simulink model "Function_Call_Subsystem_Ex"  (R2021b)
settings: Solver=VariableStepAuto  StartTime=0.0  StopTime=10.0  RelTol=1e-3
libraries: simulink x11
settings Model: Creator=t  LastModifiedBy=t

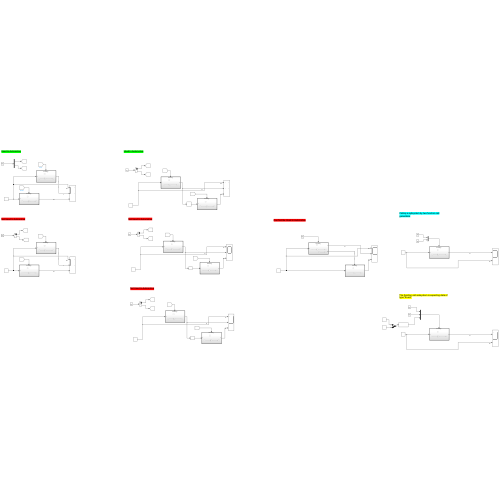
[thumbnail: Simulink's stored preview of the top-level diagram]
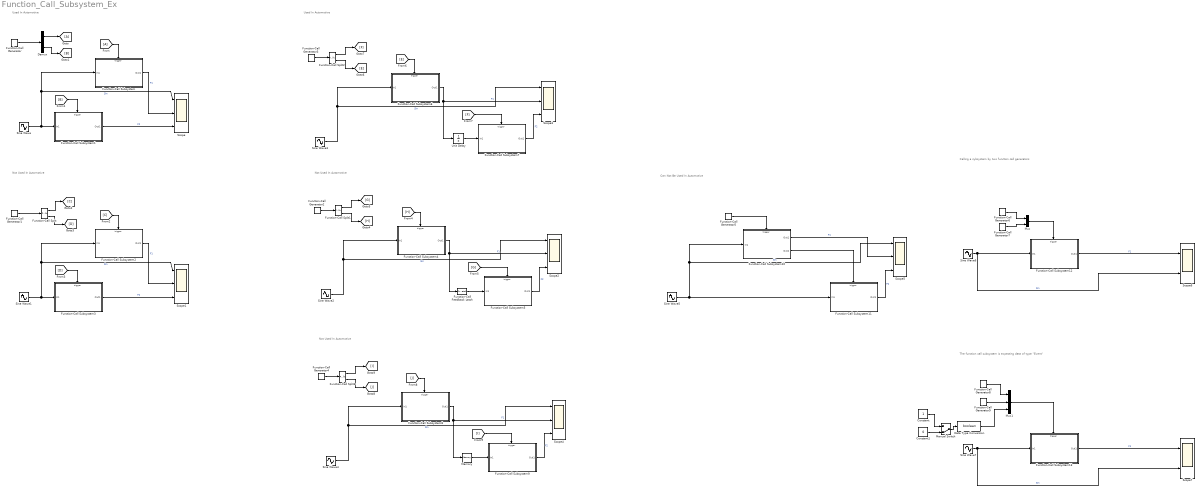
== system Function_Call_Subsystem_Ex ==
  note: Used In Automotive
  note: Not Used In Automotive
  note: Used In Automotive
  note: Not Used In Automotive
  note: Not Used In Automotive
  note: Can Not Be Used In Automotive
  note: Calling a sybsystem by two function call generators
  note: The function call subsystem is expecting data of type "Event"
  Constant : Constant
  Constant1 : Constant  Value=0
  Data Type Conversion : DataTypeConversion  OutDataTypeStr=boolean
  Demux : Demux  Outputs=2
  Function-Call Feedback Latch : FunctionCallFeedbackLatch
  Function-Call Generator{,1..6,8} (8 alike) : simulink/Ports & Subsystems/Function-Call Generator  sample_time=0.2  numberOfIterations=1  DisallowWideOutput=off
  Function-Call Generator7 : simulink/Ports & Subsystems/Function-Call Generator  sample_time=0.5  numberOfIterations=1  DisallowWideOutput=off
  Function-Call Generator9 : simulink/Ports & Subsystems/Function-Call Generator  sample_time=0.5  numberOfIterations=1  DisallowWideOutput=off
  Function-Call Split{,1..3} (4 alike) : FunctionCallSplit  IconShape=distinctive  NumOutputPorts=2  OutputPortLayout=default
  Function-Call Subsystem : Subsystem  TreatAsAtomicUnit=on
  Function-Call Subsystem1 : Subsystem  TreatAsAtomicUnit=on
  Function-Call Subsystem10 : Subsystem  TreatAsAtomicUnit=on
  Function-Call Subsystem11 : Subsystem  TreatAsAtomicUnit=on
  Function-Call Subsystem12 : Subsystem  TreatAsAtomicUnit=on
  Function-Call Subsystem13 : Subsystem  TreatAsAtomicUnit=on
  Function-Call Subsystem2 : Subsystem  TreatAsAtomicUnit=on
  Function-Call Subsystem3 : Subsystem  TreatAsAtomicUnit=on
  Function-Call Subsystem4 : Subsystem  TreatAsAtomicUnit=on
  Function-Call Subsystem5 : Subsystem  TreatAsAtomicUnit=on
  Function-Call Subsystem6 : Subsystem  TreatAsAtomicUnit=on
  Function-Call Subsystem7 : Subsystem  TreatAsAtomicUnit=on
  Function-Call Subsystem8 : Subsystem  TreatAsAtomicUnit=on
  Function-Call Subsystem9 : Subsystem  TreatAsAtomicUnit=on
  Manual Switch : ManualSwitch  CurrentSetting=0
  Memory : Memory
  Mux : Mux  Inputs=2
  Mux1 : Mux  Inputs=3
  Scope{,1..5} (6 alike) : Scope  NumInputPorts=3
  Scope6 : Scope  NumInputPorts=2
  Scope7 : Scope  NumInputPorts=2
  Sine Wave{,1..7} (8 alike) : Sin  SampleTime=0.1
  Unit Delay : UnitDelay  SampleTime=-1  HasFrameUpgradeWarning=on
  wires:
  Function-Call Generator/1 -> Demux/1
  Sine Wave/1 -> Scope/1, Function-Call Subsystem/1(In1), Function-Call Subsystem1/1(In1)  "Sin"
  Function-Call Subsystem/1(Out1) -> Scope/2  "F1"
  Function-Call Subsystem1/1(Out1) -> Scope/3  "F2"
  Demux/1 -> [A]
  Demux/2 -> [B]
  [A] -> Function-Call Subsystem/Trigger
  [B] -> Function-Call Subsystem1/Trigger
  Function-Call Subsystem3/1(Out1) -> Scope1/3  "F2"
  Function-Call Subsystem2/1(Out1) -> Scope1/2  "F1"
  Sine Wave1/1 -> Function-Call Subsystem3/1(In1), Function-Call Subsystem2/1(In1), Scope1/1  "Sin"
  Function-Call Generator1/1 -> Function-Call Split/1
  Function-Call Split/1 -> [C]
  [C] -> Function-Call Subsystem2/Trigger
  Function-Call Split/2 -> [D]
  [D] -> Function-Call Subsystem3/Trigger
  [G] -> Function-Call Subsystem5/Trigger
  [H] -> Function-Call Subsystem4/Trigger
  Function-Call Subsystem5/1(Out1) -> Scope2/3  "F2"
  Function-Call Subsystem4/1(Out1) -> Scope2/2, Function-Call Feedback Latch/1  "F1"
  Sine Wave2/1 -> Function-Call Subsystem4/1(In1), Scope2/1  "Sin"
  Function-Call Generator2/1 -> Function-Call Split1/1
  Function-Call Split1/2 -> [H]
  Function-Call Split1/1 -> [G]
  Function-Call Feedback Latch/1 -> Function-Call Subsystem5/1(In1)
  Unit Delay/1 -> Function-Call Subsystem7/1(In1)
  Function-Call Split2/1 -> [F]
  Function-Call Split2/2 -> [E]
  Function-Call Generator3/1 -> Function-Call Split2/1
  Sine Wave3/1 -> Scope3/1, Function-Call Subsystem6/1(In1)  "Sin"
  Function-Call Subsystem6/1(Out1) -> Unit Delay/1, Scope3/2  "F1"
  Function-Call Subsystem7/1(Out1) -> Scope3/3  "F2"
  [E] -> Function-Call Subsystem6/Trigger
  [F] -> Function-Call Subsystem7/Trigger
  Memory/1 -> Function-Call Subsystem9/1(In1)
  Function-Call Split3/1 -> [I]
  Function-Call Split3/2 -> [J]
  Function-Call Generator4/1 -> Function-Call Split3/1
  Sine Wave4/1 -> Scope4/1, Function-Call Subsystem8/1(In1)  "Sin"
  Function-Call Subsystem8/1(Out1) -> Memory/1, Scope4/2  "F1"
  Function-Call Subsystem9/1(Out1) -> Scope4/3  "F2"
  [J] -> Function-Call Subsystem8/Trigger
  [I] -> Function-Call Subsystem9/Trigger
  Sine Wave5/1 -> Scope5/1, Function-Call Subsystem10/1(In1), Function-Call Subsystem11/1(In1)  "Sin"
  Function-Call Subsystem10/1(Out1) -> Scope5/2  "F1"
  Function-Call Subsystem11/1(Out1) -> Scope5/3  "F2"
  Function-Call Subsystem10/2(Out2) -> Function-Call Subsystem11/Trigger
  Function-Call Generator5/1 -> Function-Call Subsystem10/Trigger
  Function-Call Subsystem12/1(Out1) -> Scope6/1  "F1"
  Sine Wave6/1 -> Scope6/2, Function-Call Subsystem12/1(In1)  "Sin"
  Function-Call Generator6/1 -> Mux/1
  Mux/1 -> Function-Call Subsystem12/Trigger
  Function-Call Generator7/1 -> Mux/2
  Function-Call Generator9/1 -> Mux1/2
  Function-Call Generator8/1 -> Mux1/1
  Sine Wave7/1 -> Function-Call Subsystem13/1(In1), Scope7/2  "Sin"
  Function-Call Subsystem13/1(Out1) -> Scope7/1  "F1"
  Mux1/1 -> Function-Call Subsystem13/Trigger
  Constant1/1 -> Manual Switch/2
  Constant/1 -> Manual Switch/1
  Manual Switch/1 -> Data Type Conversion/1
  Data Type Conversion/1 -> Mux1/3

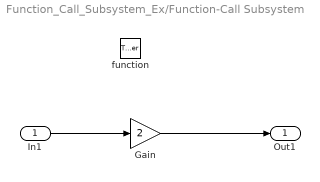
== system Function_Call_Subsystem_Ex/Function-Call Subsystem ==
  In1 : Inport
  function : TriggerPort  TriggerType=function-call  VariantControl=(inherit)
  Gain : Gain  Gain=2
  Out1 : Outport
  wires:
  In1/1 -> Gain/1
  Gain/1 -> Out1/1

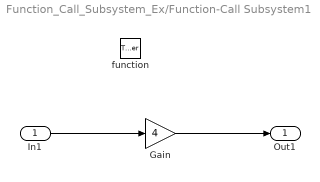
== system Function_Call_Subsystem_Ex/Function-Call Subsystem1 ==
  In1 : Inport
  function : TriggerPort  TriggerType=function-call  VariantControl=(inherit)
  Gain : Gain  Gain=4
  Out1 : Outport
  wires:
  In1/1 -> Gain/1
  Gain/1 -> Out1/1

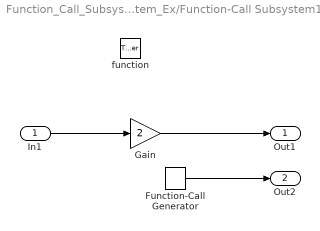
== system Function_Call_Subsystem_Ex/Function-Call Subsystem10 ==
  In1 : Inport
  function : TriggerPort  TriggerType=function-call  VariantControl=(inherit)
  Function-Call Generator : simulink/Ports & Subsystems/Function-Call Generator  sample_time=-1  numberOfIterations=1  DisallowWideOutput=off
  Gain : Gain  Gain=2
  Out1 : Outport
  Out2 : Outport  Port=2
  wires:
  In1/1 -> Gain/1
  Gain/1 -> Out1/1
  Function-Call Generator/1 -> Out2/1

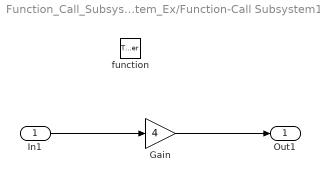
== system Function_Call_Subsystem_Ex/Function-Call Subsystem11 ==
  In1 : Inport
  function : TriggerPort  TriggerType=function-call  VariantControl=(inherit)
  Gain : Gain  Gain=4
  Out1 : Outport
  wires:
  In1/1 -> Gain/1
  Gain/1 -> Out1/1

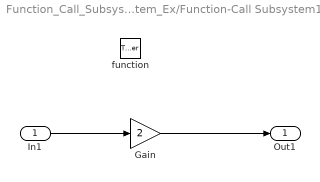
== system Function_Call_Subsystem_Ex/Function-Call Subsystem12 ==
  In1 : Inport
  function : TriggerPort  TriggerType=function-call  VariantControl=(inherit)
  Gain : Gain  Gain=2
  Out1 : Outport
  wires:
  Gain/1 -> Out1/1
  In1/1 -> Gain/1

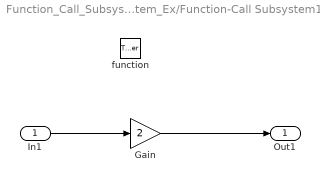
== system Function_Call_Subsystem_Ex/Function-Call Subsystem13 ==
  In1 : Inport
  function : TriggerPort  TriggerType=function-call  VariantControl=(inherit)
  Gain : Gain  Gain=2
  Out1 : Outport
  wires:
  In1/1 -> Gain/1
  Gain/1 -> Out1/1

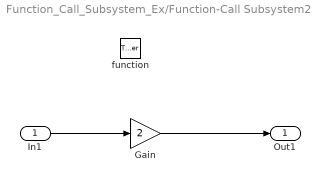
== system Function_Call_Subsystem_Ex/Function-Call Subsystem2 ==
  In1 : Inport
  function : TriggerPort  TriggerType=function-call  VariantControl=(inherit)
  Gain : Gain  Gain=2
  Out1 : Outport
  wires:
  Gain/1 -> Out1/1
  In1/1 -> Gain/1

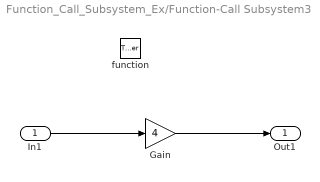
== system Function_Call_Subsystem_Ex/Function-Call Subsystem3 ==
  In1 : Inport
  function : TriggerPort  TriggerType=function-call  VariantControl=(inherit)
  Gain : Gain  Gain=4
  Out1 : Outport
  wires:
  Gain/1 -> Out1/1
  In1/1 -> Gain/1

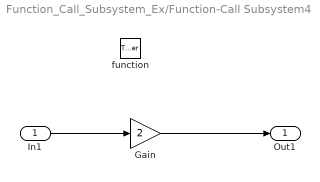
== system Function_Call_Subsystem_Ex/Function-Call Subsystem4 ==
  In1 : Inport
  function : TriggerPort  TriggerType=function-call  VariantControl=(inherit)
  Gain : Gain  Gain=2
  Out1 : Outport
  wires:
  Gain/1 -> Out1/1
  In1/1 -> Gain/1

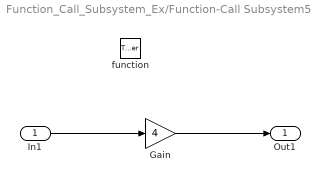
== system Function_Call_Subsystem_Ex/Function-Call Subsystem5 ==
  In1 : Inport
  function : TriggerPort  TriggerType=function-call  VariantControl=(inherit)
  Gain : Gain  Gain=4
  Out1 : Outport
  wires:
  Gain/1 -> Out1/1
  In1/1 -> Gain/1

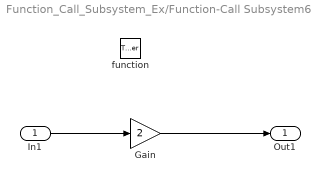
== system Function_Call_Subsystem_Ex/Function-Call Subsystem6 ==
  In1 : Inport
  function : TriggerPort  TriggerType=function-call  VariantControl=(inherit)
  Gain : Gain  Gain=2
  Out1 : Outport
  wires:
  In1/1 -> Gain/1
  Gain/1 -> Out1/1

== system Function_Call_Subsystem_Ex/Function-Call Subsystem7 ==
  In1 : Inport
  function : TriggerPort  TriggerType=function-call  VariantControl=(inherit)
  Gain : Gain  Gain=4
  Out1 : Outport
  wires:
  In1/1 -> Gain/1
  Gain/1 -> Out1/1

== system Function_Call_Subsystem_Ex/Function-Call Subsystem8 ==
  In1 : Inport
  function : TriggerPort  TriggerType=function-call  VariantControl=(inherit)
  Gain : Gain  Gain=2
  Out1 : Outport
  wires:
  In1/1 -> Gain/1
  Gain/1 -> Out1/1

== system Function_Call_Subsystem_Ex/Function-Call Subsystem9 ==
  In1 : Inport
  function : TriggerPort  TriggerType=function-call  VariantControl=(inherit)
  Gain : Gain  Gain=4
  Out1 : Outport
  wires:
  In1/1 -> Gain/1
  Gain/1 -> Out1/1
